simulink model "start_of_file_example"  (R2014a)
settings: Solver=FixedStepDiscrete  StartTime=0.0  StopTime=10.0  RelTol=1e-3
libraries: dspsigops x2, dspvision x2, simulink x2
settings Model: Creator=The MathWorks Inc.
settings DataIOCC: SaveFormat=StructureWithTime
settings OptimizationCC: ExpressionDepthLimit=2147483647
settings DebuggingCC: UnderspecifiedInitializationDetection=Classic  SolverPrmCheckMsg=none  FcnCallInpInsideContextMsg=EnableAllAsWarning  StateNameClashWarn=warning

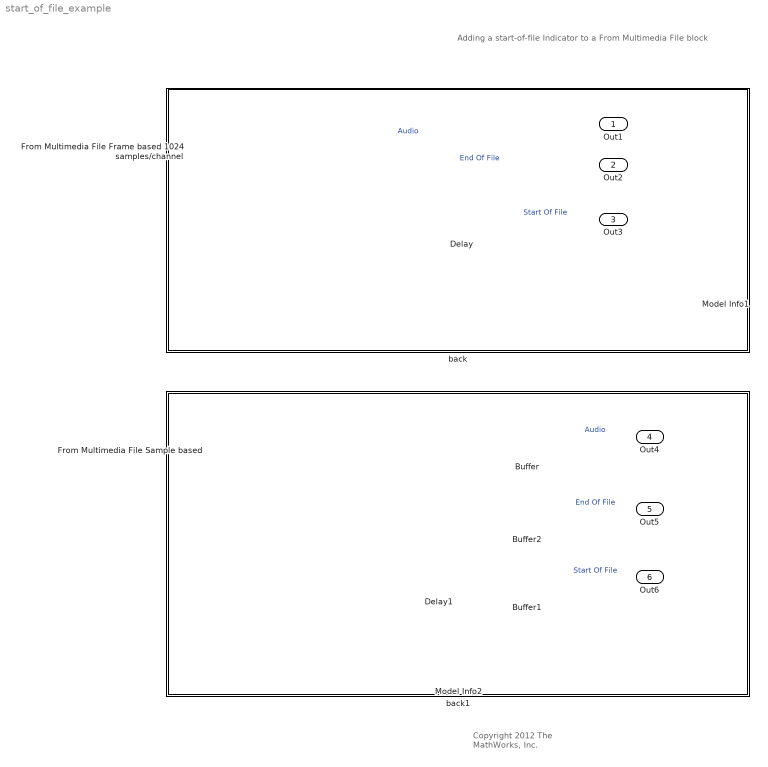
== system start_of_file_example ==
  note: Adding a start-of-file Indicator to a From Multimedia File block
  note: Copyright 2012
      | The MathWorks, Inc.
  Buffer : Buffer  N=1024  TreatMby1Signals=One channel
  Buffer1 : Buffer  N=1024  TreatMby1Signals=One channel
  Buffer2 : Buffer  N=1024  TreatMby1Signals=One channel
  Delay : dspsigops/Delay  dly_unit=Frames  delay=1  ic_detail=off  dif_ic_for_ch=off  dif_ic_for_dly=off  ic=1  reset_popup=None
  Delay1 : dspsigops/Delay  dly_unit=Frames  delay=1  ic_detail=off  dif_ic_for_ch=off  dif_ic_for_dly=off  ic=1  reset_popup=None
  From Multimedia File Frame based 1024 samples/channel : dspvision/From Multimedia File  inputFilename=speech_dft.avi  loop=on  numPlays=inf  outputStreams=Audio only  videoDataType=single  audioDataType=int16  inheritSampleTime=on  userDefinedSampleTime=1/30  noAudioOutput=off  isIntensityVideo=off  fourcc=RGB  colorVideoFormat=Separate color signals  outputEOF=on  dataOrg=Column-major  audioFrameSize=1024  computeAudioFrameSize=off  outSamplingMode=Frame based
  From Multimedia File Sample based : dspvision/From Multimedia File  inputFilename=speech_dft.avi  loop=on  numPlays=inf  outputStreams=Audio only  videoDataType=single  audioDataType=int16  inheritSampleTime=on  userDefinedSampleTime=1/30  noAudioOutput=off  isIntensityVideo=off  fourcc=RGB  colorVideoFormat=Separate color signals  outputEOF=on  dataOrg=Column-major  audioFrameSize=1  computeAudioFrameSize=off  outSamplingMode=Sample based
  Model Info1 : simulink/Model-Wide Utilities/Model Info  InitialBlockCM=None  BlockCM=None  Frame=on  DisplayStringWithTags=|  HorizontalTextAlignment=Left  LeftAlignmentValue=0.02  SourceBlockDiagram=start_of_file_example  TagMaxNumber=20
      | Restart at beginning of next frame:
      | The start-of-file indicator is the end-of-file indicator delayed by one frame.
      | The delay block initial condition is set to 1 for start-of-file at the beginning of simulation.
  Model Info2 : simulink/Model-Wide Utilities/Model Info  InitialBlockCM=None  BlockCM=None  Frame=on  DisplayStringWithTags=|  HorizontalTextAlignment=Left  LeftAlignmentValue=0.02  SourceBlockDiagram=start_of_file_example  TagMaxNumber=20
      | Restart immediately after last sample:
      | Buffer sample-based Audio. 
      | Start and end of file indicators are buffered to align with sample, not frame boundary.
  back : Subsystem
  back1 : Subsystem
  Out1 : Outport
  Out2 : Outport  Port=2
  Out3 : Outport  Port=3
  Out4 : Outport  Port=4
  Out5 : Outport  Port=5
  Out6 : Outport  Port=6
  wires:
  From Multimedia File Frame based 1024 samples/channel/1 -> Out1/1  "Audio"
  From Multimedia File Frame based 1024 samples/channel/2 -> Delay/1, Out2/1  "End Of File"
  Delay/1 -> Out3/1  "Start Of File"
  From Multimedia File Sample based/1 -> Buffer/1
  Buffer/1 -> Out4/1  "Audio"
  Buffer2/1 -> Out5/1  "End Of File"
  Buffer1/1 -> Out6/1  "Start Of File"
  Delay1/1 -> Buffer1/1
  From Multimedia File Sample based/2 -> Delay1/1, Buffer2/1

== system start_of_file_example/back ==

== system start_of_file_example/back1 ==
